simulink model "f5_VPP_controller_demo"  (R2019b)
settings: Solver=VariableStepAuto  StartTime=0.0  StopTime=6  RelTol=1e-3
settings Model: Creator=MAHMUD  LastModifiedBy=MAHMUD

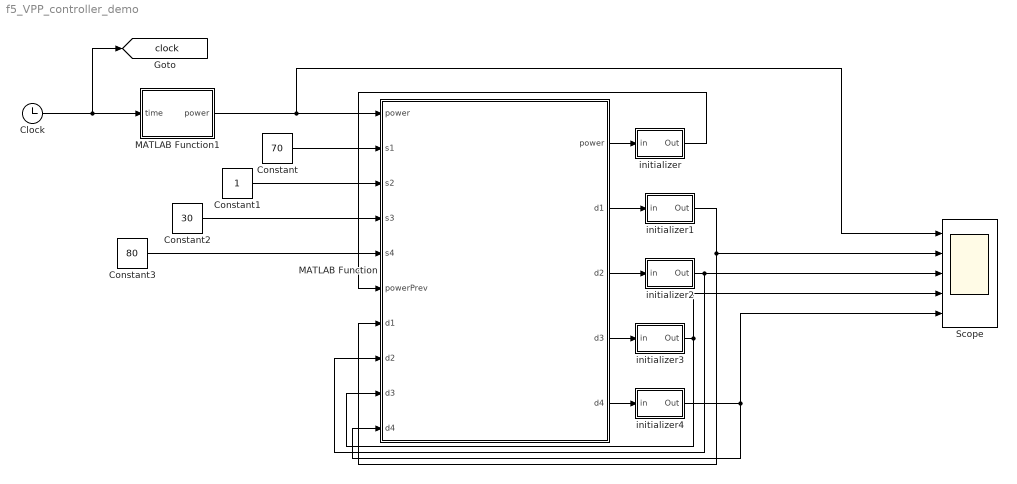
== system f5_VPP_controller_demo ==
  Clock : Clock
  Constant : Constant  Value=70
  Constant1 : Constant
  Constant2 : Constant  Value=30
  Constant3 : Constant  Value=80
  MATLAB Function : MATLAB Function  TreatAsAtomicUnit=on
  MATLAB Function1 : MATLAB Function  TreatAsAtomicUnit=on
  Scope : Scope  NumInputPorts=5
  initializer : Subsystem
  initializer1 : Subsystem
  initializer2 : Subsystem
  initializer3 : Subsystem
  initializer4 : Subsystem
  tag scope: clock=global
  wires:
  MATLAB Function1/1(power) -> Scope/1, MATLAB Function/1("power ")
  Clock/1 -> [clock], MATLAB Function1/1(time)
  Constant/1 -> MATLAB Function/2(s1)
  Constant1/1 -> MATLAB Function/3(s2)
  Constant2/1 -> MATLAB Function/4(s3)
  Constant3/1 -> MATLAB Function/5(s4)
  MATLAB Function/1(power) -> initializer/1(in)
  initializer/1(Out) -> MATLAB Function/6(powerPrev)
  MATLAB Function/2(d1) -> initializer1/1(in)
  initializer1/1(Out) -> Scope/2, MATLAB Function/7("d1 ")
  MATLAB Function/3(d2) -> initializer2/1(in)
  initializer2/1(Out) -> Scope/3, MATLAB Function/8("d2 ")
  MATLAB Function/4(d3) -> initializer3/1(in)
  initializer3/1(Out) -> Scope/4, MATLAB Function/9("d3 ")
  MATLAB Function/5(d4) -> initializer4/1(in)
  initializer4/1(Out) -> MATLAB Function/10("d4 "), Scope/5

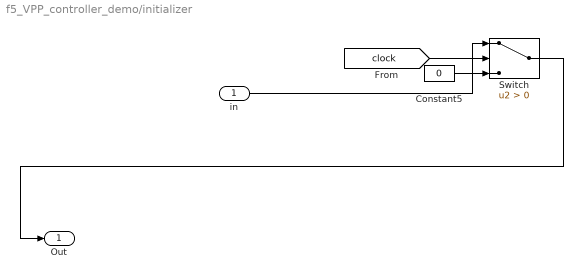
== system f5_VPP_controller_demo/initializer ==
  in : Inport
  Constant5 : Constant  Value=0
  Switch : Switch  Criteria=u2 > Threshold  ZeroCross=off
  Out : Outport
  wires:
  Constant5/1 -> Switch/3
  [clock] -> Switch/2
  in/1 -> Switch/1
  Switch/1 -> Out/1

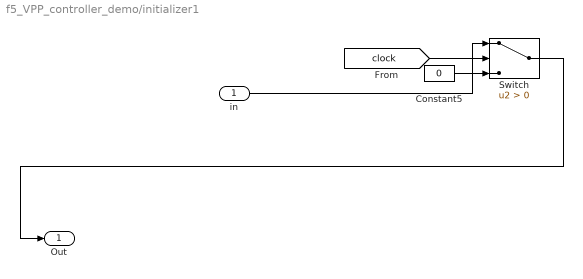
== system f5_VPP_controller_demo/initializer1 ==
  in : Inport
  Constant5 : Constant  Value=0
  Switch : Switch  Criteria=u2 > Threshold  ZeroCross=off
  Out : Outport
  wires:
  Switch/1 -> Out/1
  in/1 -> Switch/1
  [clock] -> Switch/2
  Constant5/1 -> Switch/3

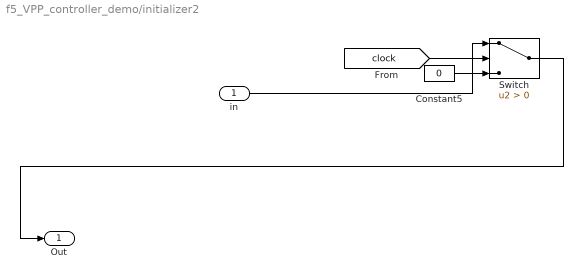
== system f5_VPP_controller_demo/initializer2 ==
  in : Inport
  Constant5 : Constant  Value=0
  Switch : Switch  Criteria=u2 > Threshold  ZeroCross=off
  Out : Outport
  wires:
  Constant5/1 -> Switch/3
  [clock] -> Switch/2
  in/1 -> Switch/1
  Switch/1 -> Out/1

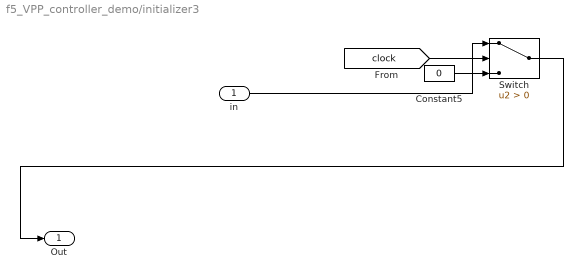
== system f5_VPP_controller_demo/initializer3 ==
  in : Inport
  Constant5 : Constant  Value=0
  Switch : Switch  Criteria=u2 > Threshold  ZeroCross=off
  Out : Outport
  wires:
  Switch/1 -> Out/1
  in/1 -> Switch/1
  [clock] -> Switch/2
  Constant5/1 -> Switch/3

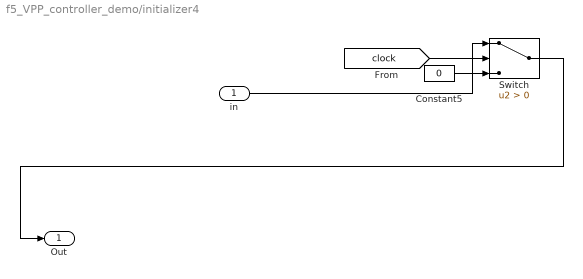
== system f5_VPP_controller_demo/initializer4 ==
  in : Inport
  Constant5 : Constant  Value=0
  Switch : Switch  Criteria=u2 > Threshold  ZeroCross=off
  Out : Outport
  wires:
  Constant5/1 -> Switch/3
  [clock] -> Switch/2
  in/1 -> Switch/1
  Switch/1 -> Out/1

== matlab function f5_VPP_controller_demo/MATLAB Function1 ==
  data: time input; power output
function power  = fcn(time)
    if time<1
        power = 21000;
    elseif time<2 
        power = 26000;
    elseif time<3
        power=30000;
    elseif time <4
        power=35000;
    elseif time <5 
        power= 27000;
    else
        power=21000;
    end

== matlab function f5_VPP_controller_demo/MATLAB Function ==
  data: power input; power output; s1 input; s2 input; s3 input; s4 input; powerPrev input; d1 input; d2 input; d3 input; d4 input; d1 output; d2 output; d3 output; d4 output
function [power,d1,d2,d3,d4] = fcn(power,s1,s2,s3,s4,powerPrev,d1,d2,d3,d4)
    if (powerPrev~=power)
        discharge=[0 0 0 0];
        soc=[s1 s2 s3 s4];
        while(power>25000)
            [m,i]=max(soc);
            soc(i)=0;
            if(m>10)
                discharge(i)=1;
                power=power-4000;
            end
        end
        d1=discharge(1);
        d2=discharge(2);
        d3=discharge(3);
        d4=discharge(4);
    end
